simulink model "dec_fir_test"  (Simulink 7.4)
settings: Solver=ode45  StartTime=0.0  StopTime=10.0  RelTol=1e-3
libraries: xbsIndex_r4 x19, casper_library_downconverter x7, casper_library_misc x1
settings Model: Creator=hong  LastModifiedBy=hong

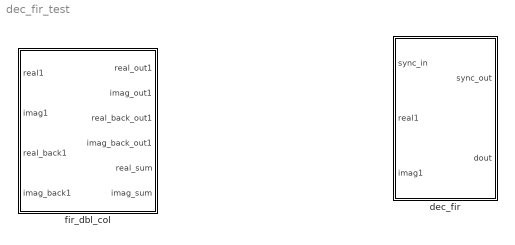
== system dec_fir_test ==
  dec_fir : Subsystem  mask(dec_fir){n_inputs=1, coeff=[1 2 3 4 5], n_bits=4, quantization=Truncate, add_latency=1, mult_latency=2, coeff_bit_width=25, coeff_bin_pt=24, adder_tree_hdl=on}
      mask prompts: n_inputs "Number of Parallel Streams"; coeff "Coefficients"; n_bits "Bit Width Out"; quantization "Quantization Behavior"; add_latency "Add Latency"; mult_latency "Mult Latency"; coeff_bit_width "Coefficient bit width"; coeff_bin_pt "Coefficient binary point"; adder_tree_hdl "Implement first stage of adder trees after multiplication as behavioural HDL"
      mask help: FIR filter which can handle multiple time samples in parallel and decimates down to 1 time sample. If coefficients are symmetric, will automatically fold before multiplying.
      settings: AttributesFormatString=|
      | 6 taps
      | 4_3 r/i
      mask Help: eval('xlWeb(''http://casper.berkeley.edu/wiki/Dec_fir'')')
      mask StyleString: edit,edit,edit,popup(Truncate|Round  (unbiased: +/- Inf)|Round  (unbiased: Even Values)),edit,edit,edit,edit,checkbox
  fir_dbl_col : Subsystem  AncestorBlock=casper_library_downconverter/fir_dbl_col  mask(fir_dbl_col){n_inputs=1, coeff=getfield( getfield( get_param( gcb,'UserData' ), 'parameters'),'coeff'), add_latency=1, mult_latency=2, coeff_bit_width=25, coeff_bin_pt=24, adder_tree_hdl=off}
      mask prompts: n_inputs "Inputs"; coeff "Coefficients"; add_latency "Add latency"; mult_latency "Mult Latency"; coeff_bit_width "Coefficient bit width"; coeff_bin_pt "Coefficient binary point"; adder_tree_hdl "Implement first stage of adder trees on output as behavioural HDL"
      mask init:
      | fir_dbl_col_init(gcb, ...
      |     'n_inputs', n_inputs, ...
      |     'coeff', coeff, ...
      |     'mult_latency', mult_latency, ...
      |     'add_latency', add_latency, ...
      |     'coeff_bit_width', coeff_bit_width, ...
      |     'coeff_bin_pt', coeff_bin_pt,  ...
      |     'adder_tree_hdl', adder_tree_hdl);
      mask Help: eval('xlWeb(''http://casper.berkeley.edu/wiki/Fir_dbl_col'')')

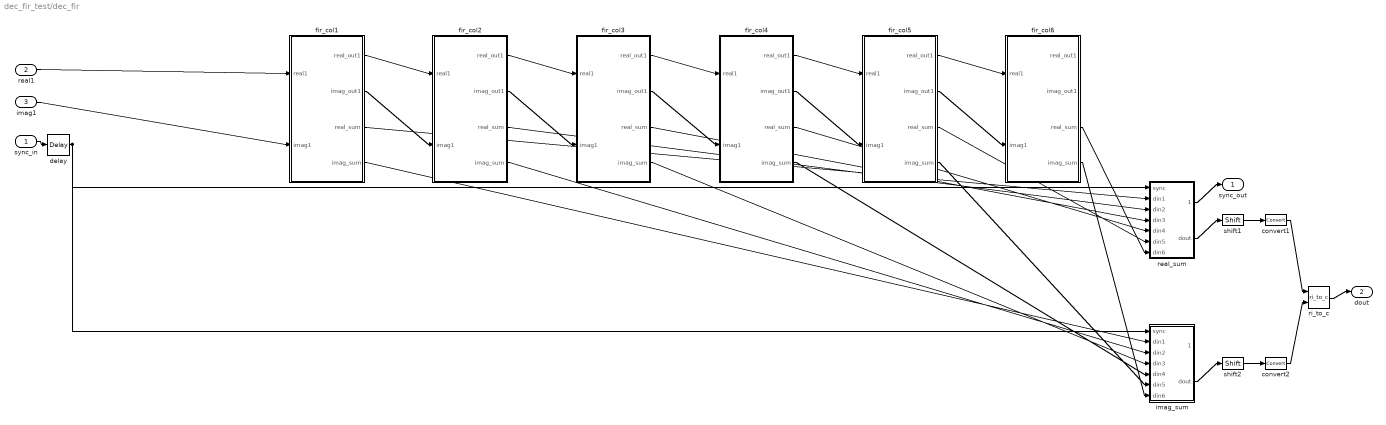
== system dec_fir_test/dec_fir ==
  sync_in : Inport
  real1 : Inport  Port=2
  imag1 : Inport  Port=3
  convert1 : xbsIndex_r4/Convert  arith_type="Signed  (2's comp)"  n_bits=4  bin_pt=3  quantization=Truncate  overflow=Wrap  latency=1  dbl_ovrd=off  pipeline=off  block_type=convert
      settings: block_version=10.1.3
  convert2 : xbsIndex_r4/Convert  arith_type="Signed  (2's comp)"  n_bits=4  bin_pt=3  quantization=Truncate  overflow=Wrap  latency=1  dbl_ovrd=off  pipeline=off  block_type=convert
      settings: block_version=10.1.3
  delay : xbsIndex_r4/Delay  en=off  latency=3  dbl_ovrd=off  reg_retiming=off  block_type=delay
  fir_col1 : Subsystem  AncestorBlock=casper_library_downconverter/fir_col  mask(fir_col){n_inputs=1, coeff=1, add_latency=1, mult_latency=2, coeff_bit_width=25, coeff_bin_pt=24, adder_tree_hdl=on}
      mask prompts: n_inputs "Inputs"; coeff "Coefficients"; add_latency "Add latency"; mult_latency "Mult Latency"; coeff_bit_width "Coefficient bit width"; coeff_bin_pt "Coefficient binary point"; adder_tree_hdl "Implement first stage of adder trees on output as behavioural HDL"
      mask Help: eval('xlWeb(''http://casper.berkeley.edu/wiki/Fir_col'')')
  fir_col2 : Subsystem  AncestorBlock=casper_library_downconverter/fir_col  mask(fir_col){n_inputs=1, coeff=2, add_latency=1, mult_latency=2, coeff_bit_width=25, coeff_bin_pt=24, adder_tree_hdl=on}
      mask prompts: n_inputs "Inputs"; coeff "Coefficients"; add_latency "Add latency"; mult_latency "Mult Latency"; coeff_bit_width "Coefficient bit width"; coeff_bin_pt "Coefficient binary point"; adder_tree_hdl "Implement first stage of adder trees on output as behavioural HDL"
      mask Help: eval('xlWeb(''http://casper.berkeley.edu/wiki/Fir_col'')')
  fir_col3 : Subsystem  AncestorBlock=casper_library_downconverter/fir_col  mask(fir_col){n_inputs=1, coeff=3, add_latency=1, mult_latency=2, coeff_bit_width=25, coeff_bin_pt=24, adder_tree_hdl=on}
      mask prompts: n_inputs "Inputs"; coeff "Coefficients"; add_latency "Add latency"; mult_latency "Mult Latency"; coeff_bit_width "Coefficient bit width"; coeff_bin_pt "Coefficient binary point"; adder_tree_hdl "Implement first stage of adder trees on output as behavioural HDL"
      mask Help: eval('xlWeb(''http://casper.berkeley.edu/wiki/Fir_col'')')
  fir_col4 : Subsystem  AncestorBlock=casper_library_downconverter/fir_col  mask(fir_col){n_inputs=1, coeff=4, add_latency=1, mult_latency=2, coeff_bit_width=25, coeff_bin_pt=24, adder_tree_hdl=on}
      mask prompts: n_inputs "Inputs"; coeff "Coefficients"; add_latency "Add latency"; mult_latency "Mult Latency"; coeff_bit_width "Coefficient bit width"; coeff_bin_pt "Coefficient binary point"; adder_tree_hdl "Implement first stage of adder trees on output as behavioural HDL"
      mask Help: eval('xlWeb(''http://casper.berkeley.edu/wiki/Fir_col'')')
  fir_col5 : Subsystem  AncestorBlock=casper_library_downconverter/fir_col  mask(fir_col){n_inputs=1, coeff=5, add_latency=1, mult_latency=2, coeff_bit_width=25, coeff_bin_pt=24, adder_tree_hdl=on}
      mask prompts: n_inputs "Inputs"; coeff "Coefficients"; add_latency "Add latency"; mult_latency "Mult Latency"; coeff_bit_width "Coefficient bit width"; coeff_bin_pt "Coefficient binary point"; adder_tree_hdl "Implement first stage of adder trees on output as behavioural HDL"
      mask Help: eval('xlWeb(''http://casper.berkeley.edu/wiki/Fir_col'')')
  fir_col6 : Subsystem  AncestorBlock=casper_library_downconverter/fir_col  mask(fir_col){n_inputs=1, coeff=6, add_latency=1, mult_latency=2, coeff_bit_width=25, coeff_bin_pt=24, adder_tree_hdl=on}
      mask prompts: n_inputs "Inputs"; coeff "Coefficients"; add_latency "Add latency"; mult_latency "Mult Latency"; coeff_bit_width "Coefficient bit width"; coeff_bin_pt "Coefficient binary point"; adder_tree_hdl "Implement first stage of adder trees on output as behavioural HDL"
      mask Help: eval('xlWeb(''http://casper.berkeley.edu/wiki/Fir_col'')')
  imag_sum : Subsystem  AncestorBlock=casper_library_misc/adder_tree  mask(adder_tree){n_inputs=6, latency=1, first_stage_hdl=off, behavioral=off}
      mask prompts: n_inputs "Number of Inputs"; latency "Add Latency"; first_stage_hdl "Use behavioural HDL for first stage of adders"; behavioral "Use behavioral HDL for all adders"
      mask help:
      | Sums all inputs using a tree of adds and delays.
      |
      | Number of inputs: The number of inputs to the block to be summed
      | Add latency: The number of clock cycles to perform one addition (affects timing).
      | Use behavioural HDL for first stage of adders: Causes the first stage of adders to be absorbed into DSP blocks if multipliers precede them (Virtex 5).
      | Use behavioural HDL for all adders: Causes all adders in all stages to be implemented in behavioural HDL (may improve timing).
      settings: AttributesFormatString=latency 3
      mask Help: eval('xlWeb(''http://casper.berkeley.edu/wiki/Adder_tree'')')
  real_sum : Subsystem  AncestorBlock=casper_library_misc/adder_tree  mask(adder_tree){n_inputs=6, latency=1, first_stage_hdl=off, behavioral=off}
      mask prompts: n_inputs "Number of Inputs"; latency "Add Latency"; first_stage_hdl "Use behavioural HDL for first stage of adders"; behavioral "Use behavioral HDL for all adders"
      mask help:
      | Sums all inputs using a tree of adds and delays.
      |
      | Number of inputs: The number of inputs to the block to be summed
      | Add latency: The number of clock cycles to perform one addition (affects timing).
      | Use behavioural HDL for first stage of adders: Causes the first stage of adders to be absorbed into DSP blocks if multipliers precede them (Virtex 5).
      | Use behavioural HDL for all adders: Causes all adders in all stages to be implemented in behavioural HDL (may improve timing).
      settings: AttributesFormatString=latency 3
      mask Help: eval('xlWeb(''http://casper.berkeley.edu/wiki/Adder_tree'')')
  ri_to_c : casper_library_misc/ri_to_c  SystemSampleTime=-1
  shift1 : xbsIndex_r4/Shift  shift_dir=Left  shift_bits=1  en=off  latency=0  precision=Full  arith_type="Signed  (2's comp)"  n_bits=16  bin_pt=14  quantization=Truncate  overflow=Wrap  dbl_ovrd=off  block_type=shift
      settings: block_version=10.1.3
  shift2 : xbsIndex_r4/Shift  shift_dir=Left  shift_bits=1  en=off  latency=0  precision=Full  arith_type="Signed  (2's comp)"  n_bits=16  bin_pt=14  quantization=Truncate  overflow=Wrap  dbl_ovrd=off  block_type=shift
      settings: block_version=10.1.3
  sync_out : Outport
  dout : Outport  Port=2
  wires:
  real1/1 -> fir_col1/1(real1)
  imag1/1 -> fir_col1/2(imag1)
  fir_col1/3(real_sum) -> real_sum/2(din1)
  fir_col1/4(imag_sum) -> imag_sum/2(din1)
  fir_col1/1(real_out1) -> fir_col2/1(real1)
  fir_col1/2(imag_out1) -> fir_col2/2(imag1)
  fir_col2/3(real_sum) -> real_sum/3(din2)
  fir_col2/4(imag_sum) -> imag_sum/3(din2)
  fir_col2/1(real_out1) -> fir_col3/1(real1)
  fir_col2/2(imag_out1) -> fir_col3/2(imag1)
  fir_col3/3(real_sum) -> real_sum/4(din3)
  fir_col3/4(imag_sum) -> imag_sum/4(din3)
  fir_col3/1(real_out1) -> fir_col4/1(real1)
  fir_col3/2(imag_out1) -> fir_col4/2(imag1)
  fir_col4/3(real_sum) -> real_sum/5(din4)
  fir_col4/4(imag_sum) -> imag_sum/5(din4)
  fir_col4/1(real_out1) -> fir_col5/1(real1)
  fir_col4/2(imag_out1) -> fir_col5/2(imag1)
  fir_col5/3(real_sum) -> real_sum/6(din5)
  fir_col5/4(imag_sum) -> imag_sum/6(din5)
  fir_col5/1(real_out1) -> fir_col6/1(real1)
  fir_col5/2(imag_out1) -> fir_col6/2(imag1)
  fir_col6/3(real_sum) -> real_sum/7(din6)
  fir_col6/4(imag_sum) -> imag_sum/7(din6)
  real_sum/2(dout) -> shift1/1
  imag_sum/2(dout) -> shift2/1
  shift1/1 -> convert1/1
  shift2/1 -> convert2/1
  convert1/1 -> ri_to_c/1
  convert2/1 -> ri_to_c/2
  ri_to_c/1 -> dout/1
  sync_in/1 -> delay/1
  delay/1 -> real_sum/1(sync), imag_sum/1(sync)
  real_sum/1(sync_out) -> sync_out/1

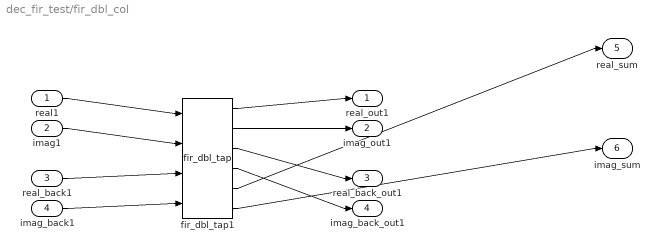
== system dec_fir_test/fir_dbl_col ==
  real1 : Inport
  imag1 : Inport  Port=2
  real_back1 : Inport  Port=3
  imag_back1 : Inport  Port=4
  fir_dbl_tap1 : casper_library_downconverter/fir_dbl_tap  SystemSampleTime=-1  factor=0.1  add_latency=1  mult_latency=2  coeff_bit_width=25  coeff_bin_pt=24
  real_out1 : Outport
  imag_out1 : Outport  Port=2
  real_back_out1 : Outport  Port=3
  imag_back_out1 : Outport  Port=4
  real_sum : Outport  Port=5
  imag_sum : Outport  Port=6
  wires:
  real1/1 -> fir_dbl_tap1/1
  imag1/1 -> fir_dbl_tap1/2
  real_back1/1 -> fir_dbl_tap1/3
  imag_back1/1 -> fir_dbl_tap1/4
  fir_dbl_tap1/1 -> real_out1/1
  fir_dbl_tap1/2 -> imag_out1/1
  fir_dbl_tap1/3 -> real_back_out1/1
  fir_dbl_tap1/4 -> imag_back_out1/1
  fir_dbl_tap1/5 -> real_sum/1
  fir_dbl_tap1/6 -> imag_sum/1

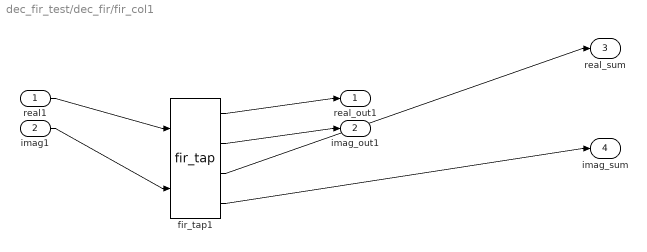
== system dec_fir_test/dec_fir/fir_col1 ==
  real1 : Inport
  imag1 : Inport  Port=2
  fir_tap1 : casper_library_downconverter/fir_tap  SystemSampleTime=-1  factor=1  latency=2  coeff_bit_width=25  coeff_bin_pt=24
  real_out1 : Outport
  imag_out1 : Outport  Port=2
  real_sum : Outport  Port=3
  imag_sum : Outport  Port=4
  wires:
  real1/1 -> fir_tap1/1
  imag1/1 -> fir_tap1/2
  fir_tap1/1 -> real_out1/1
  fir_tap1/2 -> imag_out1/1
  fir_tap1/3 -> real_sum/1
  fir_tap1/4 -> imag_sum/1

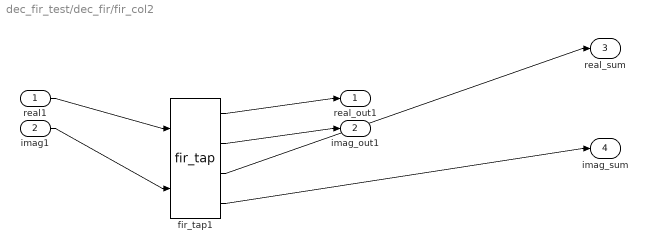
== system dec_fir_test/dec_fir/fir_col2 ==
  real1 : Inport
  imag1 : Inport  Port=2
  fir_tap1 : casper_library_downconverter/fir_tap  SystemSampleTime=-1  factor=2  latency=2  coeff_bit_width=25  coeff_bin_pt=24
  real_out1 : Outport
  imag_out1 : Outport  Port=2
  real_sum : Outport  Port=3
  imag_sum : Outport  Port=4
  wires:
  real1/1 -> fir_tap1/1
  imag1/1 -> fir_tap1/2
  fir_tap1/1 -> real_out1/1
  fir_tap1/2 -> imag_out1/1
  fir_tap1/3 -> real_sum/1
  fir_tap1/4 -> imag_sum/1

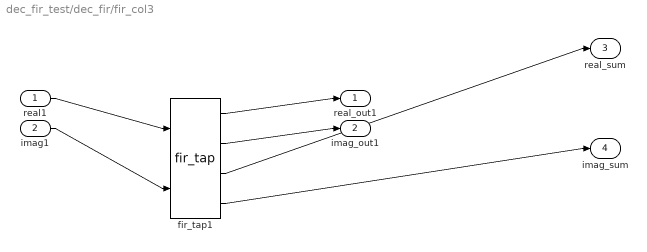
== system dec_fir_test/dec_fir/fir_col3 ==
  real1 : Inport
  imag1 : Inport  Port=2
  fir_tap1 : casper_library_downconverter/fir_tap  SystemSampleTime=-1  factor=3  latency=2  coeff_bit_width=25  coeff_bin_pt=24
  real_out1 : Outport
  imag_out1 : Outport  Port=2
  real_sum : Outport  Port=3
  imag_sum : Outport  Port=4
  wires:
  real1/1 -> fir_tap1/1
  imag1/1 -> fir_tap1/2
  fir_tap1/1 -> real_out1/1
  fir_tap1/2 -> imag_out1/1
  fir_tap1/3 -> real_sum/1
  fir_tap1/4 -> imag_sum/1

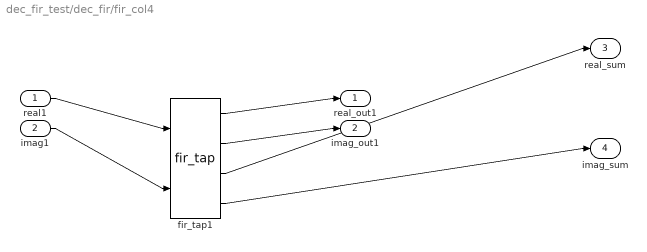
== system dec_fir_test/dec_fir/fir_col4 ==
  real1 : Inport
  imag1 : Inport  Port=2
  fir_tap1 : casper_library_downconverter/fir_tap  SystemSampleTime=-1  factor=4  latency=2  coeff_bit_width=25  coeff_bin_pt=24
  real_out1 : Outport
  imag_out1 : Outport  Port=2
  real_sum : Outport  Port=3
  imag_sum : Outport  Port=4
  wires:
  real1/1 -> fir_tap1/1
  imag1/1 -> fir_tap1/2
  fir_tap1/1 -> real_out1/1
  fir_tap1/2 -> imag_out1/1
  fir_tap1/3 -> real_sum/1
  fir_tap1/4 -> imag_sum/1

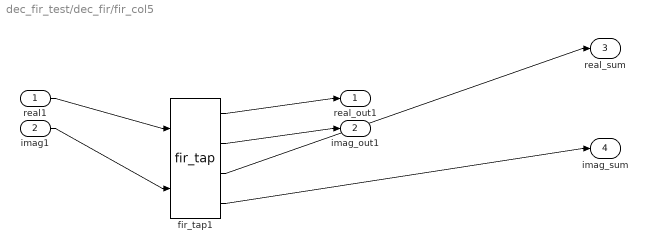
== system dec_fir_test/dec_fir/fir_col5 ==
  real1 : Inport
  imag1 : Inport  Port=2
  fir_tap1 : casper_library_downconverter/fir_tap  SystemSampleTime=-1  factor=5  latency=2  coeff_bit_width=25  coeff_bin_pt=24
  real_out1 : Outport
  imag_out1 : Outport  Port=2
  real_sum : Outport  Port=3
  imag_sum : Outport  Port=4
  wires:
  real1/1 -> fir_tap1/1
  imag1/1 -> fir_tap1/2
  fir_tap1/1 -> real_out1/1
  fir_tap1/2 -> imag_out1/1
  fir_tap1/3 -> real_sum/1
  fir_tap1/4 -> imag_sum/1

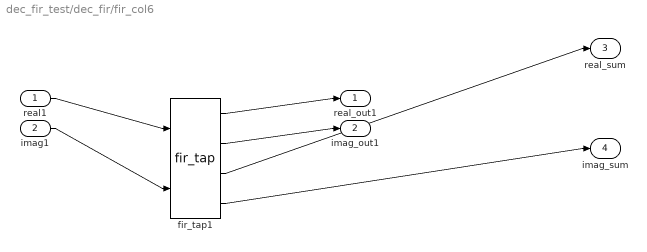
== system dec_fir_test/dec_fir/fir_col6 ==
  real1 : Inport
  imag1 : Inport  Port=2
  fir_tap1 : casper_library_downconverter/fir_tap  SystemSampleTime=-1  factor=6  latency=2  coeff_bit_width=25  coeff_bin_pt=24
  real_out1 : Outport
  imag_out1 : Outport  Port=2
  real_sum : Outport  Port=3
  imag_sum : Outport  Port=4
  wires:
  real1/1 -> fir_tap1/1
  imag1/1 -> fir_tap1/2
  fir_tap1/1 -> real_out1/1
  fir_tap1/2 -> imag_out1/1
  fir_tap1/3 -> real_sum/1
  fir_tap1/4 -> imag_sum/1

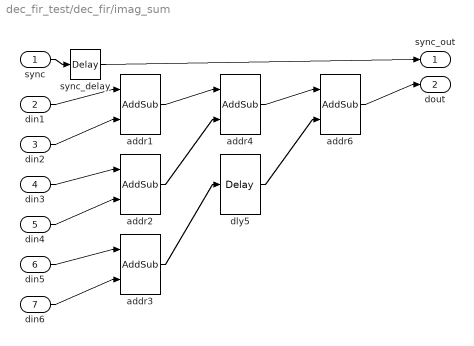
== system dec_fir_test/dec_fir/imag_sum ==
  sync : Inport
  din1 : Inport  Port=2
  din2 : Inport  Port=3
  din3 : Inport  Port=4
  din4 : Inport  Port=5
  din5 : Inport  Port=6
  din6 : Inport  Port=7
  addr{1..4,6} (5 alike) : xbsIndex_r4/AddSub  mode=Addition  use_carryin=off  use_carryout=off  en=off  latency=1  precision=Full  arith_type=Unsigned  n_bits=16  bin_pt=14  quantization=Truncate  overflow=Wrap  dbl_ovrd=off  use_behavioral_HDL=off  hw_selection=Fabric  pipelined=on  use_rpm=on  block_type=addsub
      addr1 settings: block_version=10.1.3
      addr3 settings: block_version=10.1.3
  dly5 : xbsIndex_r4/Delay  en=off  latency=1  dbl_ovrd=off  reg_retiming=on  block_type=delay
      settings: block_version=11.4
  sync_delay : xbsIndex_r4/Delay  en=off  latency=3  dbl_ovrd=off  reg_retiming=on  block_type=delay
  sync_out : Outport
  dout : Outport  Port=2
  wires:
  sync/1 -> sync_delay/1
  sync_delay/1 -> sync_out/1
  din1/1 -> addr1/1
  din2/1 -> addr1/2
  din3/1 -> addr2/1
  din4/1 -> addr2/2
  din5/1 -> addr3/1
  din6/1 -> addr3/2
  addr1/1 -> addr4/1
  addr2/1 -> addr4/2
  addr3/1 -> dly5/1
  addr4/1 -> addr6/1
  dly5/1 -> addr6/2
  addr6/1 -> dout/1

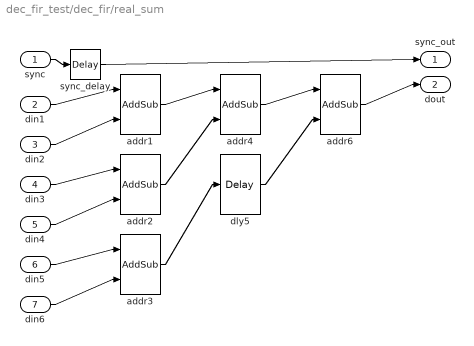
== system dec_fir_test/dec_fir/real_sum ==
  sync : Inport
  din1 : Inport  Port=2
  din2 : Inport  Port=3
  din3 : Inport  Port=4
  din4 : Inport  Port=5
  din5 : Inport  Port=6
  din6 : Inport  Port=7
  addr{1..4,6} (5 alike) : xbsIndex_r4/AddSub  mode=Addition  use_carryin=off  use_carryout=off  en=off  latency=1  precision=Full  arith_type=Unsigned  n_bits=16  bin_pt=14  quantization=Truncate  overflow=Wrap  dbl_ovrd=off  use_behavioral_HDL=off  hw_selection=Fabric  pipelined=on  use_rpm=on  block_type=addsub
      addr1 settings: block_version=10.1.3
      addr3 settings: block_version=10.1.3
  dly5 : xbsIndex_r4/Delay  en=off  latency=1  dbl_ovrd=off  reg_retiming=on  block_type=delay
      settings: block_version=11.4
  sync_delay : xbsIndex_r4/Delay  en=off  latency=3  dbl_ovrd=off  reg_retiming=on  block_type=delay
  sync_out : Outport
  dout : Outport  Port=2
  wires:
  sync/1 -> sync_delay/1
  sync_delay/1 -> sync_out/1
  din1/1 -> addr1/1
  din2/1 -> addr1/2
  din3/1 -> addr2/1
  din4/1 -> addr2/2
  din5/1 -> addr3/1
  din6/1 -> addr3/2
  addr1/1 -> addr4/1
  addr2/1 -> addr4/2
  addr3/1 -> dly5/1
  addr4/1 -> addr6/1
  dly5/1 -> addr6/2
  addr6/1 -> dout/1
